simulink model "ptp_servo"  (R2026a)
settings: Solver=FixedStepDiscrete  StopTime=P.T_stop  FixedStep=P.Ts
values from neighbouring files (symbols this model uses):
  P = ptp_params()    [run_servo_model.m]
undefined symbols (not defined in the file or in its folder): DiscIntNeverNeededParam
settings Model: Creator=srikarvelavarthipati  LastModifiedBy=srikarvelavarthipati

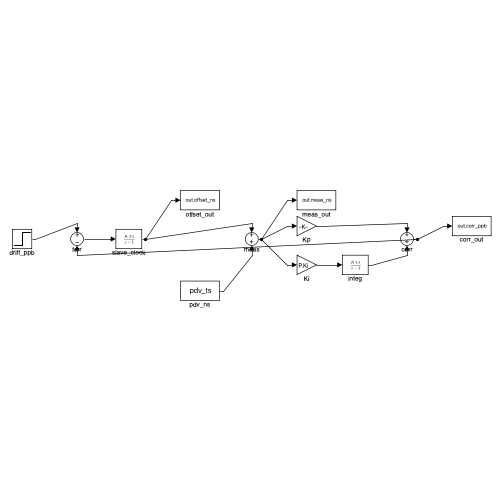
[thumbnail: Simulink's stored preview of the top-level diagram]
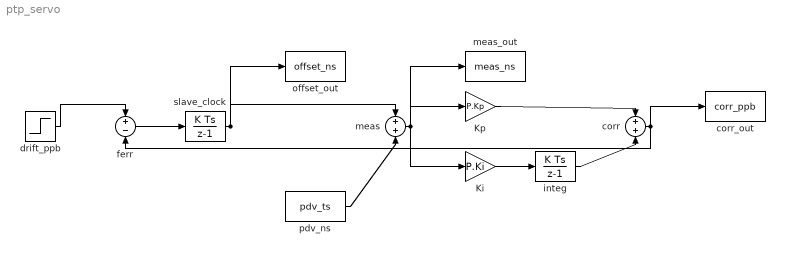
== system ptp_servo ==
  Ki : Gain  Gain=P.Ki
  Kp : Gain  Gain=P.Kp
  corr : Sum
  corr_out : ToWorkspace  VariableName=corr_ppb  SampleTime=P.Ts
  drift_ppb : Step  Time=P.drift_step_k*P.Ts  InitialValue=P.drift_ppb  FinalValue=P.drift_ppb + P.drift_step_ppb  SampleTime=P.Ts
  ferr : Sum  Inputs=+-
  integ : DiscreteIntegrator  gainval=1  SampleTime=P.Ts  ICPrevOutput=DiscIntNeverNeededParam  ICPrevScaledInput=DiscIntNeverNeededParam
  meas : Sum
  meas_out : ToWorkspace  VariableName=meas_ns  SampleTime=P.Ts
  offset_out : ToWorkspace  VariableName=offset_ns  SampleTime=P.Ts
  pdv_ns : FromWorkspace  VariableName=pdv_ts  SampleTime=P.Ts  Interpolate=off  OutputAfterFinalValue=Holding final value
  slave_clock : DiscreteIntegrator  gainval=1  InitialCondition=P.init_offset_sim_ns  SampleTime=P.Ts  ICPrevOutput=DiscIntNeverNeededParam  ICPrevScaledInput=DiscIntNeverNeededParam
  wires:
  drift_ppb/1 -> ferr/1
  ferr/1 -> slave_clock/1
  slave_clock/1 -> meas/1, offset_out/1
  pdv_ns/1 -> meas/2
  meas/1 -> Kp/1, Ki/1, meas_out/1
  Ki/1 -> integ/1
  Kp/1 -> corr/1
  integ/1 -> corr/2
  corr/1 -> ferr/2, corr_out/1
